simulink model "vesselPowerCert"  (R2026a)
settings: Solver=FixedStepDiscrete  StopTime=115200  FixedStep=60
model workspace (MAT data in the model file):
  VAR_ESS = 2
  VAR_GEN = 2
  VAR_PROP_ARCH = 3
  VAR_SHORE = 2
  capEnergy_kWh = 60
  capPower_kW = 2500
  designSpeed_kn = 14
  dpBase_kW = 1250
  dpRippleAmp_kW = 480
  dt_s = 60
  essEnergy_kWh = 1200
  essEtaRT = 0.92
  essPower_kW = 1500
  essSocInit = 0.65
  etaDrive = 0.97
  etaGearbox = 0.97
  etaMotor = 0.96
  etaShaftMach = 0.95
  genLoadMax = 0.9
  genSfocLoadOpt = 0.8
  genSfocMin = 192
  genUnitPower_kW = 1800
  hotelTab_kW = [550 605 550 880 550 605 550]
  mePower_kW = 5200
  meSfocLoadOpt = 0.85
  meSfocMin = 178
  modeTab = [1 2 3 4 3 2 1]
  propPower_kW = 4800
  seaMargin = 0.06
  seaTab = [0 1 3 4 3 1 0]
  shorePower_kW = 1600
  tBreak_s = [0 14400 18000 46800 68400 97200 100800]
  vTab_kn = [0 6 14 0 12 6 0]
settings Model: Creator=KoayXianCong  LastModifiedBy=KoayXianCong

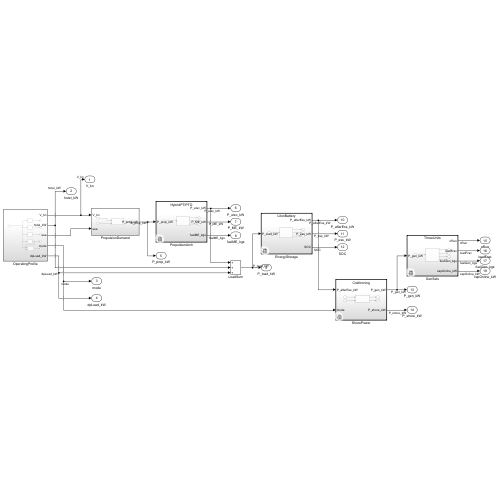
[thumbnail: Simulink's stored preview of the top-level diagram]
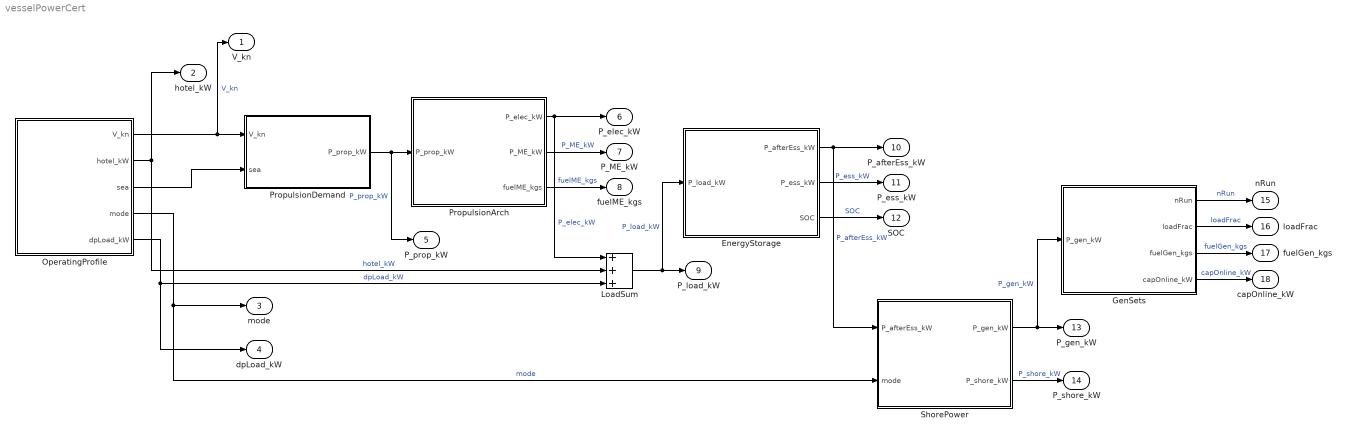
== system vesselPowerCert ==
  EnergyStorage : Subsystem  Variant=on  VariantActivationTime=startup
  GenSets : Subsystem  Variant=on  VariantActivationTime=startup
  LoadSum : Sum  Inputs=+++
  OperatingProfile : Subsystem
  PropulsionArch : Subsystem  Variant=on  VariantActivationTime=startup
  PropulsionDemand : Subsystem
  ShorePower : Subsystem  Variant=on  VariantActivationTime=startup
  V_kn : Outport
  hotel_kW : Outport  Port=2
  mode : Outport  Port=3
  dpLoad_kW : Outport  Port=4
  P_prop_kW : Outport  Port=5
  P_elec_kW : Outport  Port=6
  P_ME_kW : Outport  Port=7
  fuelME_kgs : Outport  Port=8
  P_load_kW : Outport  Port=9
  P_afterEss_kW : Outport  Port=10
  P_ess_kW : Outport  Port=11
  SOC : Outport  Port=12
  P_gen_kW : Outport  Port=13
  P_shore_kW : Outport  Port=14
  nRun : Outport  Port=15
  loadFrac : Outport  Port=16
  fuelGen_kgs : Outport  Port=17
  capOnline_kW : Outport  Port=18
  wires:
  PropulsionDemand/1(P_prop_kW) -> PropulsionArch/1(P_prop_kW), P_prop_kW/1  "P_prop_kW"
  OperatingProfile/2(hotel_kW) -> hotel_kW/1, LoadSum/2  "hotel_kW"
  OperatingProfile/1(V_kn) -> V_kn/1, PropulsionDemand/1(V_kn)  "V_kn"
  OperatingProfile/3(sea) -> PropulsionDemand/2(sea)
  OperatingProfile/5(dpLoad_kW) -> LoadSum/3, dpLoad_kW/1  "dpLoad_kW"
  OperatingProfile/4(mode) -> ShorePower/2(mode), mode/1  "mode"
  PropulsionArch/2(P_ME_kW) -> P_ME_kW/1  "P_ME_kW"
  PropulsionArch/1(P_elec_kW) -> LoadSum/1, P_elec_kW/1  "P_elec_kW"
  EnergyStorage/2(P_ess_kW) -> P_ess_kW/1  "P_ess_kW"
  PropulsionArch/3(fuelME_kgs) -> fuelME_kgs/1  "fuelME_kgs"
  GenSets/1(nRun) -> nRun/1  "nRun"
  LoadSum/1 -> P_load_kW/1, EnergyStorage/1(P_load_kW)  "P_load_kW"
  EnergyStorage/1(P_afterEss_kW) -> ShorePower/1(P_afterEss_kW), P_afterEss_kW/1  "P_afterEss_kW"
  EnergyStorage/3(SOC) -> SOC/1  "SOC"
  ShorePower/1(P_gen_kW) -> GenSets/1(P_gen_kW), P_gen_kW/1  "P_gen_kW"
  GenSets/3(fuelGen_kgs) -> fuelGen_kgs/1  "fuelGen_kgs"
  ShorePower/2(P_shore_kW) -> P_shore_kW/1  "P_shore_kW"
  GenSets/2(loadFrac) -> loadFrac/1  "loadFrac"
  GenSets/4(capOnline_kW) -> capOnline_kW/1  "capOnline_kW"

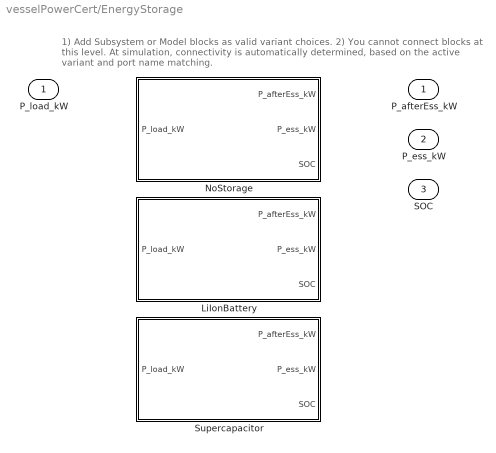
== system vesselPowerCert/EnergyStorage ==
  note: 1) Add Subsystem or Model blocks as valid variant choices.
      | 2) You cannot connect blocks at this level. At simulation, connectivity is automatically
      | determined, based on the active variant and port name matching.
  P_load_kW : Inport
  LiIonBattery : Subsystem  TreatAsAtomicUnit=on  VariantControl=VAR_ESS==2
  NoStorage : Subsystem  TreatAsAtomicUnit=on  VariantControl=VAR_ESS==1
  Supercapacitor : Subsystem  TreatAsAtomicUnit=on  VariantControl=VAR_ESS==3
  P_afterEss_kW : Outport
  P_ess_kW : Outport  Port=2
  SOC : Outport  Port=3

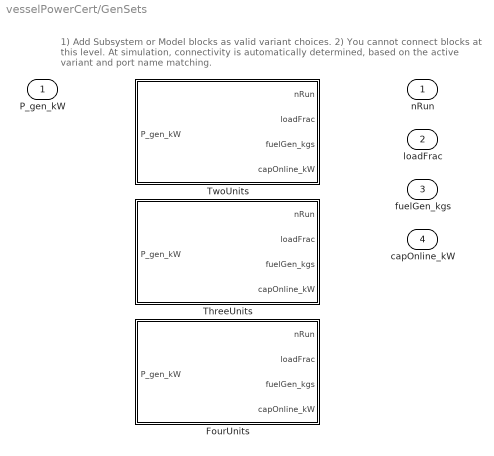
== system vesselPowerCert/GenSets ==
  note: 1) Add Subsystem or Model blocks as valid variant choices.
      | 2) You cannot connect blocks at this level. At simulation, connectivity is automatically
      | determined, based on the active variant and port name matching.
  P_gen_kW : Inport
  FourUnits : Subsystem  TreatAsAtomicUnit=on  VariantControl=VAR_GEN==3
  ThreeUnits : Subsystem  TreatAsAtomicUnit=on  VariantControl=VAR_GEN==2
  TwoUnits : Subsystem  TreatAsAtomicUnit=on  VariantControl=VAR_GEN==1
  nRun : Outport
  loadFrac : Outport  Port=2
  fuelGen_kgs : Outport  Port=3
  capOnline_kW : Outport  Port=4

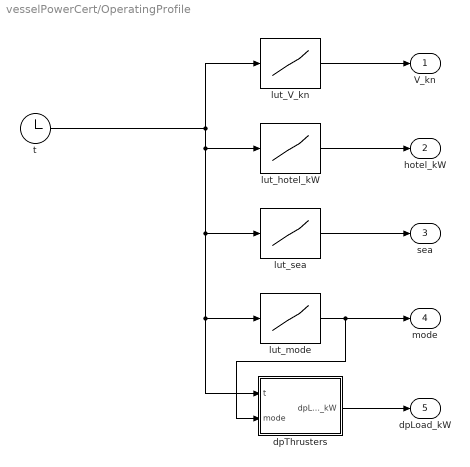
== system vesselPowerCert/OperatingProfile ==
  dpThrusters : MATLAB Function  TreatAsAtomicUnit=on
  lut_V_kn : Lookup_n-D  NumberOfTableDimensions=1  BreakpointsForDimension1=tBreak_s  Table=vTab_kn  InterpMethod=Flat  ExtrapMethod=Clip  InternalRulePriority=Speed  RndMeth=Simplest
  lut_hotel_kW : Lookup_n-D  NumberOfTableDimensions=1  BreakpointsForDimension1=tBreak_s  Table=hotelTab_kW  InterpMethod=Flat  ExtrapMethod=Clip  InternalRulePriority=Speed  RndMeth=Simplest
  lut_mode : Lookup_n-D  NumberOfTableDimensions=1  BreakpointsForDimension1=tBreak_s  Table=modeTab  InterpMethod=Flat  ExtrapMethod=Clip  InternalRulePriority=Speed  RndMeth=Simplest
  lut_sea : Lookup_n-D  NumberOfTableDimensions=1  BreakpointsForDimension1=tBreak_s  Table=seaTab  InterpMethod=Flat  ExtrapMethod=Clip  InternalRulePriority=Speed  RndMeth=Simplest
  t : Clock
  V_kn : Outport
  hotel_kW : Outport  Port=2
  sea : Outport  Port=3
  mode : Outport  Port=4
  dpLoad_kW : Outport  Port=5
  wires:
  t/1 -> dpThrusters/1(t), lut_mode/1, lut_sea/1, lut_hotel_kW/1, lut_V_kn/1
  lut_V_kn/1 -> V_kn/1
  lut_hotel_kW/1 -> hotel_kW/1
  lut_sea/1 -> sea/1
  lut_mode/1 -> dpThrusters/2(mode), mode/1
  dpThrusters/1(dpLoad_kW) -> dpLoad_kW/1

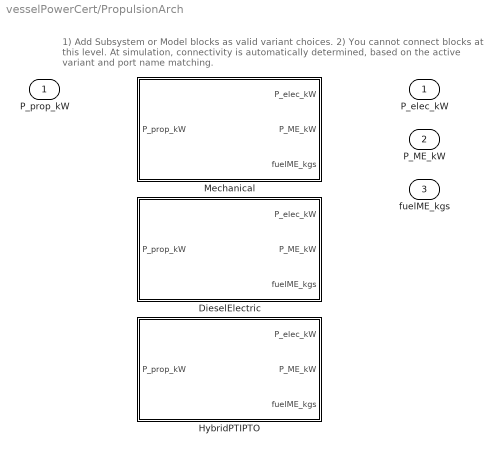
== system vesselPowerCert/PropulsionArch ==
  note: 1) Add Subsystem or Model blocks as valid variant choices.
      | 2) You cannot connect blocks at this level. At simulation, connectivity is automatically
      | determined, based on the active variant and port name matching.
  P_prop_kW : Inport
  DieselElectric : Subsystem  TreatAsAtomicUnit=on  VariantControl=VAR_PROP_ARCH==2
  HybridPTIPTO : Subsystem  TreatAsAtomicUnit=on  VariantControl=VAR_PROP_ARCH==3
  Mechanical : Subsystem  TreatAsAtomicUnit=on  VariantControl=VAR_PROP_ARCH==1
  P_elec_kW : Outport
  P_ME_kW : Outport  Port=2
  fuelME_kgs : Outport  Port=3

== system vesselPowerCert/PropulsionDemand ==
  V_kn : Inport
  sea : Inport  Port=2
  fcn : MATLAB Function  TreatAsAtomicUnit=on
  P_prop_kW : Outport
  wires:
  V_kn/1 -> fcn/1(V_kn)
  sea/1 -> fcn/2(sea)
  fcn/1(P_prop_kW) -> P_prop_kW/1

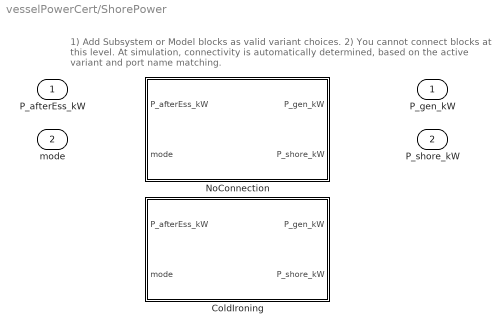
== system vesselPowerCert/ShorePower ==
  note: 1) Add Subsystem or Model blocks as valid variant choices.
      | 2) You cannot connect blocks at this level. At simulation, connectivity is automatically
      | determined, based on the active variant and port name matching.
  P_afterEss_kW : Inport
  mode : Inport  Port=2
  ColdIroning : Subsystem  TreatAsAtomicUnit=on  VariantControl=VAR_SHORE==2
  NoConnection : Subsystem  TreatAsAtomicUnit=on  VariantControl=VAR_SHORE==1
  P_gen_kW : Outport
  P_shore_kW : Outport  Port=2

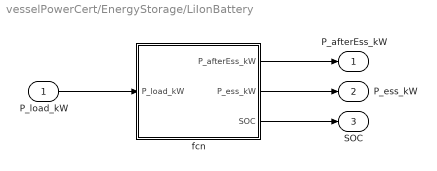
== system vesselPowerCert/EnergyStorage/LiIonBattery ==
  P_load_kW : Inport
  fcn : MATLAB Function  TreatAsAtomicUnit=on
  P_afterEss_kW : Outport
  P_ess_kW : Outport  Port=2
  SOC : Outport  Port=3
  wires:
  P_load_kW/1 -> fcn/1(P_load_kW)
  fcn/1(P_afterEss_kW) -> P_afterEss_kW/1
  fcn/2(P_ess_kW) -> P_ess_kW/1
  fcn/3(SOC) -> SOC/1

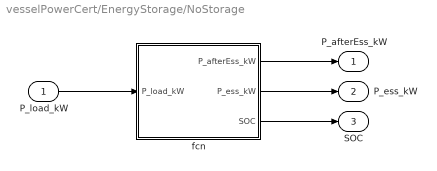
== system vesselPowerCert/EnergyStorage/NoStorage ==
  P_load_kW : Inport
  fcn : MATLAB Function  TreatAsAtomicUnit=on
  P_afterEss_kW : Outport
  P_ess_kW : Outport  Port=2
  SOC : Outport  Port=3
  wires:
  P_load_kW/1 -> fcn/1(P_load_kW)
  fcn/1(P_afterEss_kW) -> P_afterEss_kW/1
  fcn/2(P_ess_kW) -> P_ess_kW/1
  fcn/3(SOC) -> SOC/1

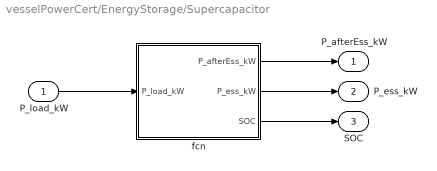
== system vesselPowerCert/EnergyStorage/Supercapacitor ==
  P_load_kW : Inport
  fcn : MATLAB Function  TreatAsAtomicUnit=on
  P_afterEss_kW : Outport
  P_ess_kW : Outport  Port=2
  SOC : Outport  Port=3
  wires:
  P_load_kW/1 -> fcn/1(P_load_kW)
  fcn/1(P_afterEss_kW) -> P_afterEss_kW/1
  fcn/2(P_ess_kW) -> P_ess_kW/1
  fcn/3(SOC) -> SOC/1

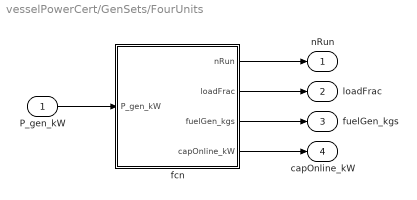
== system vesselPowerCert/GenSets/FourUnits ==
  P_gen_kW : Inport
  fcn : MATLAB Function  TreatAsAtomicUnit=on
  nRun : Outport
  loadFrac : Outport  Port=2
  fuelGen_kgs : Outport  Port=3
  capOnline_kW : Outport  Port=4
  wires:
  P_gen_kW/1 -> fcn/1(P_gen_kW)
  fcn/1(nRun) -> nRun/1
  fcn/2(loadFrac) -> loadFrac/1
  fcn/3(fuelGen_kgs) -> fuelGen_kgs/1
  fcn/4(capOnline_kW) -> capOnline_kW/1

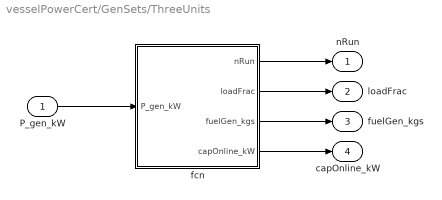
== system vesselPowerCert/GenSets/ThreeUnits ==
  P_gen_kW : Inport
  fcn : MATLAB Function  TreatAsAtomicUnit=on
  nRun : Outport
  loadFrac : Outport  Port=2
  fuelGen_kgs : Outport  Port=3
  capOnline_kW : Outport  Port=4
  wires:
  P_gen_kW/1 -> fcn/1(P_gen_kW)
  fcn/1(nRun) -> nRun/1
  fcn/2(loadFrac) -> loadFrac/1
  fcn/3(fuelGen_kgs) -> fuelGen_kgs/1
  fcn/4(capOnline_kW) -> capOnline_kW/1

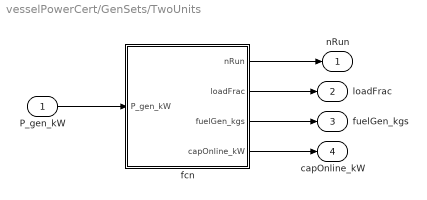
== system vesselPowerCert/GenSets/TwoUnits ==
  P_gen_kW : Inport
  fcn : MATLAB Function  TreatAsAtomicUnit=on
  nRun : Outport
  loadFrac : Outport  Port=2
  fuelGen_kgs : Outport  Port=3
  capOnline_kW : Outport  Port=4
  wires:
  P_gen_kW/1 -> fcn/1(P_gen_kW)
  fcn/1(nRun) -> nRun/1
  fcn/2(loadFrac) -> loadFrac/1
  fcn/3(fuelGen_kgs) -> fuelGen_kgs/1
  fcn/4(capOnline_kW) -> capOnline_kW/1

== system vesselPowerCert/PropulsionArch/DieselElectric ==
  P_prop_kW : Inport
  fcn : MATLAB Function  TreatAsAtomicUnit=on
  P_elec_kW : Outport
  P_ME_kW : Outport  Port=2
  fuelME_kgs : Outport  Port=3
  wires:
  P_prop_kW/1 -> fcn/1(P_prop_kW)
  fcn/1(P_elec_kW) -> P_elec_kW/1
  fcn/2(P_ME_kW) -> P_ME_kW/1
  fcn/3(fuelME_kgs) -> fuelME_kgs/1

== system vesselPowerCert/PropulsionArch/HybridPTIPTO ==
  P_prop_kW : Inport
  fcn : MATLAB Function  TreatAsAtomicUnit=on
  P_elec_kW : Outport
  P_ME_kW : Outport  Port=2
  fuelME_kgs : Outport  Port=3
  wires:
  P_prop_kW/1 -> fcn/1(P_prop_kW)
  fcn/1(P_elec_kW) -> P_elec_kW/1
  fcn/2(P_ME_kW) -> P_ME_kW/1
  fcn/3(fuelME_kgs) -> fuelME_kgs/1

== system vesselPowerCert/PropulsionArch/Mechanical ==
  P_prop_kW : Inport
  fcn : MATLAB Function  TreatAsAtomicUnit=on
  P_elec_kW : Outport
  P_ME_kW : Outport  Port=2
  fuelME_kgs : Outport  Port=3
  wires:
  P_prop_kW/1 -> fcn/1(P_prop_kW)
  fcn/1(P_elec_kW) -> P_elec_kW/1
  fcn/2(P_ME_kW) -> P_ME_kW/1
  fcn/3(fuelME_kgs) -> fuelME_kgs/1

== system vesselPowerCert/ShorePower/ColdIroning ==
  P_afterEss_kW : Inport
  mode : Inport  Port=2
  fcn : MATLAB Function  TreatAsAtomicUnit=on
  P_gen_kW : Outport
  P_shore_kW : Outport  Port=2
  wires:
  P_afterEss_kW/1 -> fcn/1(P_afterEss_kW)
  mode/1 -> fcn/2(mode)
  fcn/1(P_gen_kW) -> P_gen_kW/1
  fcn/2(P_shore_kW) -> P_shore_kW/1

== system vesselPowerCert/ShorePower/NoConnection ==
  P_afterEss_kW : Inport
  mode : Inport  Port=2
  fcn : MATLAB Function  TreatAsAtomicUnit=on
  P_gen_kW : Outport
  P_shore_kW : Outport  Port=2
  wires:
  P_afterEss_kW/1 -> fcn/1(P_afterEss_kW)
  mode/1 -> fcn/2(mode)
  fcn/1(P_gen_kW) -> P_gen_kW/1
  fcn/2(P_shore_kW) -> P_shore_kW/1

== matlab function vesselPowerCert/EnergyStorage/NoStorage/fcn ==
  data: P_load_kW input; P_afterEss_kW output; P_ess_kW output; SOC output; essSocInit parameter; essPower_kW parameter; essEnergy_kWh parameter; essEtaRT parameter; capPower_kW parameter; capEnergy_kWh parameter; dt_s parameter
function [P_afterEss_kW, P_ess_kW, SOC] = fcn(P_load_kW, essSocInit, essPower_kW, essEnergy_kWh, essEtaRT, capPower_kW, capEnergy_kWh, dt_s)
% No energy storage fitted - the plant follows the load exactly.
P_afterEss_kW = P_load_kW;
P_ess_kW      = 0;
SOC           = 0;

== matlab function vesselPowerCert/EnergyStorage/LiIonBattery/fcn ==
  data: P_load_kW input; P_afterEss_kW output; P_ess_kW output; SOC output; essSocInit parameter; essPower_kW parameter; essEnergy_kWh parameter; essEtaRT parameter; capPower_kW parameter; capEnergy_kWh parameter; dt_s parameter
function [P_afterEss_kW, P_ess_kW, SOC] = fcn(P_load_kW, essSocInit, essPower_kW, essEnergy_kWh, essEtaRT, capPower_kW, capEnergy_kWh, dt_s)
% Li-ion battery shaving peaks against a 15 minute moving average, which is
% long enough to let the generators sit at a steady operating point.
persistent soc pavg
if isempty(soc)
    soc  = essSocInit;
    pavg = P_load_kW;
end
a    = dt_s / (900 + dt_s);
pavg = pavg + a * (P_load_kW - pavg);
[soc, P_ess_kW] = vpcEssStep(soc, P_load_kW, pavg, essPower_kW, ...
                             essEnergy_kWh, essEtaRT, dt_s);
P_afterEss_kW = P_load_kW - P_ess_kW;
SOC = soc;

== matlab function vesselPowerCert/EnergyStorage/Supercapacitor/fcn ==
  data: P_load_kW input; P_afterEss_kW output; P_ess_kW output; SOC output; essSocInit parameter; essPower_kW parameter; essEnergy_kWh parameter; essEtaRT parameter; capPower_kW parameter; capEnergy_kWh parameter; dt_s parameter
function [P_afterEss_kW, P_ess_kW, SOC] = fcn(P_load_kW, essSocInit, essPower_kW, essEnergy_kWh, essEtaRT, capPower_kW, capEnergy_kWh, dt_s)
% Supercapacitor: little energy but high power, so it only rides out fast
% transients against a 2 minute average.
persistent soc pavg
if isempty(soc)
    soc  = 0.6;
    pavg = P_load_kW;
end
a    = dt_s / (120 + dt_s);
pavg = pavg + a * (P_load_kW - pavg);
[soc, P_ess_kW] = vpcEssStep(soc, P_load_kW, pavg, capPower_kW, ...
                             capEnergy_kWh, 0.97, dt_s);
P_afterEss_kW = P_load_kW - P_ess_kW;
SOC = soc;

== matlab function vesselPowerCert/GenSets/TwoUnits/fcn ==
  data: P_gen_kW input; nRun output; loadFrac output; fuelGen_kgs output; capOnline_kW output; genUnitPower_kW parameter; genLoadMax parameter; genSfocMin parameter; genSfocLoadOpt parameter
function [nRun, loadFrac, fuelGen_kgs, capOnline_kW] = fcn(P_gen_kW, genUnitPower_kW, genLoadMax, genSfocMin, genSfocLoadOpt)
% Two diesel generator sets with equal load sharing.
nInstalled = 2;
[nRun, loadFrac, fuelGen_kgs, capOnline_kW] = vpcGenDispatch( ...
    P_gen_kW, nInstalled, genUnitPower_kW, genLoadMax, ...
    genSfocMin, genSfocLoadOpt);

== matlab function vesselPowerCert/PropulsionDemand/fcn ==
  data: V_kn input; P_prop_kW output; sea input; designSpeed_kn parameter; propPower_kW parameter; seaMargin parameter
function P_prop_kW = fcn(V_kn, sea, designSpeed_kn, propPower_kW, seaMargin)
% Admiralty-style cubic speed-power law plus a sea-state margin.
vRatio  = V_kn / max(designSpeed_kn, 1e-6);
P_calm  = propPower_kW * vRatio^3;
P_prop_kW = P_calm * (1 + seaMargin * sea);

== matlab function vesselPowerCert/GenSets/ThreeUnits/fcn ==
  data: P_gen_kW input; nRun output; loadFrac output; fuelGen_kgs output; capOnline_kW output; genUnitPower_kW parameter; genLoadMax parameter; genSfocMin parameter; genSfocLoadOpt parameter
function [nRun, loadFrac, fuelGen_kgs, capOnline_kW] = fcn(P_gen_kW, genUnitPower_kW, genLoadMax, genSfocMin, genSfocLoadOpt)
% Three diesel generator sets with equal load sharing.
nInstalled = 3;
[nRun, loadFrac, fuelGen_kgs, capOnline_kW] = vpcGenDispatch( ...
    P_gen_kW, nInstalled, genUnitPower_kW, genLoadMax, ...
    genSfocMin, genSfocLoadOpt);

== matlab function vesselPowerCert/GenSets/FourUnits/fcn ==
  data: P_gen_kW input; nRun output; loadFrac output; fuelGen_kgs output; capOnline_kW output; genUnitPower_kW parameter; genLoadMax parameter; genSfocMin parameter; genSfocLoadOpt parameter
function [nRun, loadFrac, fuelGen_kgs, capOnline_kW] = fcn(P_gen_kW, genUnitPower_kW, genLoadMax, genSfocMin, genSfocLoadOpt)
% Four diesel generator sets with equal load sharing.
nInstalled = 4;
[nRun, loadFrac, fuelGen_kgs, capOnline_kW] = vpcGenDispatch( ...
    P_gen_kW, nInstalled, genUnitPower_kW, genLoadMax, ...
    genSfocMin, genSfocLoadOpt);

== matlab function vesselPowerCert/OperatingProfile/dpThrusters ==
  data: t input; dpLoad_kW output; mode input; dpBase_kW parameter; dpRippleAmp_kW parameter
function dpLoad_kW = fcn(t, mode, dpBase_kW, dpRippleAmp_kW)
% Thruster demand while station keeping, zero otherwise.
if mode > 3.5
    ripple = dpRippleAmp_kW * (sin(2*pi*t/600) + 0.5*sin(2*pi*t/1500));
    dpLoad_kW = max(0, dpBase_kW + ripple);
else
    dpLoad_kW = 0;
end

== matlab function vesselPowerCert/PropulsionArch/Mechanical/fcn ==
  data: P_prop_kW input; P_elec_kW output; P_ME_kW output; fuelME_kgs output; etaGearbox parameter; etaDrive parameter; etaMotor parameter; etaShaftMach parameter; mePower_kW parameter; meSfocMin parameter; meSfocLoadOpt parameter
function [P_elec_kW, P_ME_kW, fuelME_kgs] = fcn(P_prop_kW, etaGearbox, etaDrive, etaMotor, etaShaftMach, mePower_kW, meSfocMin, meSfocLoadOpt)
% Direct mechanical drive: the main engine carries all propulsion through
% the gearbox, and the generators see only the hotel load.
P_elec_kW  = 0;
P_ME_kW    = P_prop_kW / etaGearbox;
fuelME_kgs = vpcSfoc(P_ME_kW, mePower_kW, meSfocMin, meSfocLoadOpt);

== matlab function vesselPowerCert/PropulsionArch/DieselElectric/fcn ==
  data: P_prop_kW input; P_elec_kW output; P_ME_kW output; fuelME_kgs output; etaGearbox parameter; etaDrive parameter; etaMotor parameter; etaShaftMach parameter; mePower_kW parameter; meSfocMin parameter; meSfocLoadOpt parameter
function [P_elec_kW, P_ME_kW, fuelME_kgs] = fcn(P_prop_kW, etaGearbox, etaDrive, etaMotor, etaShaftMach, mePower_kW, meSfocMin, meSfocLoadOpt)
% Diesel-electric: no main engine at all - propulsion becomes an
% electrical load behind the converter and motor.
P_elec_kW  = P_prop_kW / (etaDrive * etaMotor);
P_ME_kW    = 0;
fuelME_kgs = 0;

== matlab function vesselPowerCert/PropulsionArch/HybridPTIPTO/fcn ==
  data: P_prop_kW input; P_elec_kW output; P_ME_kW output; fuelME_kgs output; etaGearbox parameter; etaDrive parameter; etaMotor parameter; etaShaftMach parameter; mePower_kW parameter; meSfocMin parameter; meSfocLoadOpt parameter
function [P_elec_kW, P_ME_kW, fuelME_kgs] = fcn(P_prop_kW, etaGearbox, etaDrive, etaMotor, etaShaftMach, mePower_kW, meSfocMin, meSfocLoadOpt)
% Hybrid PTI/PTO: hold the main engine near its best-SFOC point and let the
% shaft machine take up the difference as motor (PTI) or generator (PTO).
P_ME_best  = mePower_kW * meSfocLoadOpt;
P_shaft    = min(P_prop_kW, P_ME_best);
P_deficit  = max(0, P_prop_kW - P_shaft);
P_elec_kW  = P_deficit / (etaShaftMach * etaDrive);
P_ME_kW    = P_shaft / etaGearbox;
fuelME_kgs = vpcSfoc(P_ME_kW, mePower_kW, meSfocMin, meSfocLoadOpt);

== matlab function vesselPowerCert/ShorePower/NoConnection/fcn ==
  data: P_afterEss_kW input; P_gen_kW output; mode input; P_shore_kW output; shorePower_kW parameter
function [P_gen_kW, P_shore_kW] = fcn(P_afterEss_kW, mode, shorePower_kW)
% No shore connection: the vessel always supplies its own load.
P_gen_kW   = P_afterEss_kW;
P_shore_kW = 0;

== matlab function vesselPowerCert/ShorePower/ColdIroning/fcn ==
  data: P_afterEss_kW input; P_gen_kW output; mode input; P_shore_kW output; shorePower_kW parameter
function [P_gen_kW, P_shore_kW] = fcn(P_afterEss_kW, mode, shorePower_kW)
% Cold ironing: alongside in harbour (mode 1) the shore supply carries the
% load up to the rating of the connection; any excess falls to the plant.
if mode < 1.5
    P_shore_kW = min(max(P_afterEss_kW,0), shorePower_kW);
    P_gen_kW   = P_afterEss_kW - P_shore_kW;
else
    P_shore_kW = 0;
    P_gen_kW   = P_afterEss_kW;
end
